simulink model "pmsm_foc_drive"  (R2021b)
settings: Solver=daessc  StartTime=0.0  StopTime=0.2  MaxStep=1e-3  RelTol=1e-3  AbsTol=1e-3  EnableMultiTasking=on
PreLoadFcn:
  | SystemParams;
StopFcn:
  | ee_addSimlogTimeStamp(bdroot)
undefined symbols (not defined in the file): ControllerParams, PmsmParams, SensorParams, TestScenarioParams
libraries: fl_lib x12, nesl_utility x8, ee_lib x2, spsFirstOrderFilterLib x1, simulink_extras x1
Description:
  | PMSM Drive Using Field-Oriented Control.
  | Copyright 2021 The MathWorks, Inc.
settings Model: Creator=agonzale  LastModifiedBy=agonzale
settings SolverCC: AutoScaleAbsTol=off  AlgebraicLoopSolver=TrustRegion
settings DataIOCC: LimitDataPoints=on  MaxDataPoints=10000
settings OptimizationCC: LifeSpan=inf
settings DebuggingCC: AllowSymbolicDim=off  SFUnexpectedBacktrackingDiag=warning  SFNoUnconditionalDefaultTransitionDiag=warning  SFExecutionAtInitializationDiag=none  SFMachineParentedDataDiag=warning  ArithmeticOperatorsInVariantConditions=warning
settings SFSimCC: SimUseLocalCustomCode=off  CustomCodeUndefinedFunction=UseInterfaceOnly
settings RTWCC: RTWUseLocalCustomCode=off
settings CodeAppCC: StateflowObjectComments=on
settings GRTTargetCC: TargetLangStandard=C89/C90 (ANSI)
settings ConfigComp: CovMetricSettings=dw  CovSaveCumulativeToWorkspaceVar=on  CovSaveSingleToWorkspaceVar=on  CovExternalEMLEnable=off  CovSFcnEnable=off
settings SimscapeCC: SimscapeLogType=all  SimscapeLogSimulationStatistics=on  SimscapeLogName=simlog_pmsm_foc_drive  SimscapeLogLimitData=off  SimscapeLogDataHistory=10000

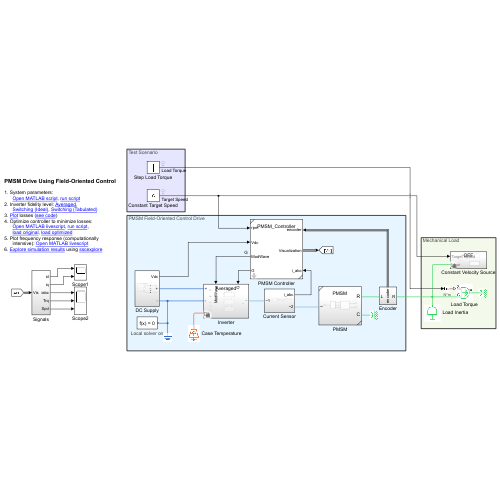
[thumbnail: Simulink's stored preview of the top-level diagram]
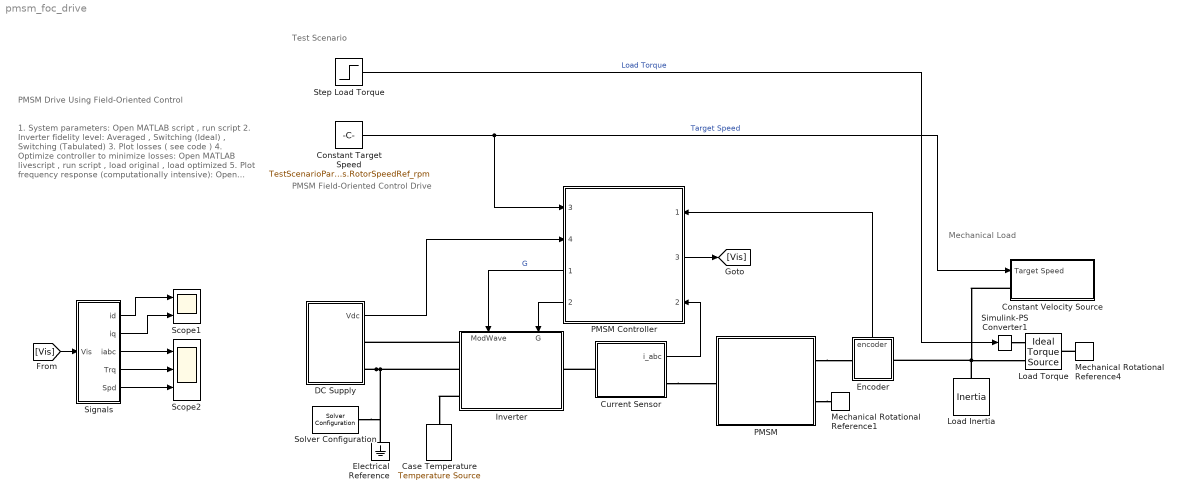
== system pmsm_foc_drive ==
  note: Mechanical Load
  note: PMSM Field-Oriented Control Drive
  note: Test Scenario
  note: 1. System parameters:
      | Open MATLAB script , run script
      | 2. Inverter fidelity level: Averaged ,
      | Switching (Ideal) , Switching (Tabulated)
      | 3. Plot losses ( see code )
      | 4. Optimize controller to minimize losses:
      | Open MATLAB livescript , run script ,
      | load original , load optimized
      | 5. Plot frequency response (computationally
      | intensive): Open MATLAB livescript
      | 6. Explore simulation results using sscexplore
  note: PMSM Drive Using Field-Oriented Control
  Case Temperature : fl_lib/Thermal/Thermal Sources/Temperature Source  temperature=InverterParams.TemperatureCase degC
  Constant Target Speed : Constant  Value=TestScenarioParams.RotorSpeedRef_rpm  SampleTime=ControllerParams.SampleTime
  Constant Velocity Source : Subsystem  Variant=on  VariantControlMode=label  LabelModeActiveChoice=OFF
  Current Sensor : Subsystem
  DC Supply : Subsystem
  Electrical Reference : fl_lib/Electrical/Electrical Elements/Electrical Reference
  Encoder : Subsystem
      settings: PortSchema="{\"entries\":[{\"content\":{\"sides\":[{\"content\":{\"connectorIds\":[\"LConn1\"]},\"type\":\"ConnectorPlacement.EquallySpacedRectSide\",\"uuid\":\"cfad22f7-4ca5-4e38-a161-f69c3faf7447\"},{\"content\":{\"connectorIds\":[\"RConn1\"],\"side\":\"RIGHT\"},\"type\":\"ConnectorPlacement.EquallySpacedRectSide\",\"uuid\":\"720e2ecf-f383-4111-97af-41d99d9b093d\"},{\"content\":{\"connectorIds\":[\"Out1\"],\"side\":\"TOP\"},\"type\":\"ConnectorPlacement.EquallySpacedRectSide\",\"uuid\":\"072894f0-fc0d-4f40-82e8-543eb6144e32\"}]},\"type\":\"ConnectorPlacement.EquallySpacedConnector\",\"uuid\":\"8d289e27-8023-447e-8610-dc73c3ce1339\"}],\"packageUris\":[\"http://schema.mathworks.com/mf0/Connector/R2020b\"],\"version\":\"1.0\"}"
  Inverter : Subsystem  Variant=on  VariantControlMode=label  VariantControl=Choice  LabelModeActiveChoice=Averaged
      settings: PortSchema="{\"entries\":[{\"content\":{\"sides\":[{\"content\":{\"connectorIds\":[\"LConn1\",\"LConn2\",\"LConn3\"]},\"type\":\"ConnectorPlacement.EquallySpacedRectSide\",\"uuid\":\"a5731130-aa3c-45df-b5d7-9e85c7611628\"},{\"content\":{\"connectorIds\":[\"RConn1\"],\"side\":\"RIGHT\"},\"type\":\"ConnectorPlacement.EquallySpacedRectSide\",\"uuid\":\"36730f5a-16d9-4cf3-b45d-c3a376589b1d\"},{\"content\":{\"connectorIds\":[\"In1\",\"In2\"],\"side\":\"TOP\"},\"type\":\"ConnectorPlacement.EquallySpacedRectSide\",\"uuid\":\"1e8f061d-b5bb-4e2a-be7e-dfb277e3f506\"}]},\"type\":\"ConnectorPlacement.EquallySpacedConnector\",\"uuid\":\"5a1efd64-0ec3-4b0f-b9d9-80575f7546cb\"}],\"packageUris\":[\"http://schema.mathworks.com/mf0/Connector/R2020b\"],\"version\":\"1.0\"}"
  Load Inertia : fl_lib/Mechanical/Rotational Elements/Inertia  inertia=MechLoadParams.Inertia kg*m^2  num_ports=foundation.enum.numPorts2.one  w_specify=on  w_priority=None  w=0 rpm  w_nominal_specify=off  w_nominal_unit=rad/s  w_nominal_value=1  t_specify=off  t_priority=None  t=0 N*m  t_nominal_specify=off  t_nominal_unit=N*m  t_nominal_value=1
  Load Torque : fl_lib/Mechanical/Mechanical Sources/Ideal Torque Source
  Mechanical Rotational Reference1 : fl_lib/Mechanical/Rotational Elements/Mechanical Rotational Reference
  Mechanical Rotational Reference4 : fl_lib/Mechanical/Rotational Elements/Mechanical Rotational Reference
  PMSM : Subsystem  ReferencedSubsystem=PMSM
  PMSM Controller : Subsystem  VariantControl=Averaged  ReferencedSubsystem=PMSM_Controller  ControllerParameters=ControllerParams
      settings: PortSchema="{\"entries\":[{\"content\":{\"sides\":[{\"content\":{\"connectorIds\":[\"In1\",\"Out3\",\"In2\"]},\"type\":\"ConnectorPlacement.EquallySpacedRectSide\",\"uuid\":\"4c32f1a4-bd89-4f05-8eaa-e2dd24abb257\"},{\"content\":{\"connectorIds\":[\"In3\",\"In4\",\"Out1\",\"Out2\"],\"side\":\"RIGHT\"},\"type\":\"ConnectorPlacement.EquallySpacedRectSide\",\"uuid\":\"3a536089-b16f-4be7-9641-6e190c11a3d2\"},{\"content\":{\"connectorIds\":[],\"side\":\"TOP\"},\"type\":\"ConnectorPlacement.EquallySpacedRectSide\",\"uuid\":\"a2701a3e-e366-4020-97eb-8b06a1d4835f\"}]},\"type\":\"ConnectorPlacement.EquallySpacedConnector\",\"uuid\":\"63f34eb4-489c-429c-82ff-74daaf150fe3\"}],\"packageUris\":[\"http://schema.mathworks.com/mf0/Connector/R2020b\"],\"version\":\"1.0\"}"
  Scope1 : Scope  NumInputPorts=2
  Scope2 : Scope  NumInputPorts=3
  "Signals " : Subsystem
  Simulink-PS Converter1 : nesl_utility/Simulink-PS Converter  PhysicalDomain=network_engine_domain  SubClassName=ps_input  LeftPortType=input  RightPortType=output  PseudoPeriodic=off  Frequencies=[]  NoiseDistribution=none  NoiseParameters=[]  Unit=N*m  AffineConversion=off  FilteringAndDerivatives=provide  SimscapeFilterOrder=1  InputFilterTimeConstant=0.001  UdotUserProvided=0
      settings: SourceProductBaseCode=PW,SS
  Solver Configuration : nesl_utility/Solver Configuration  Tag=ModelFeatures  PhysicalDomain=network_engine_domain  SubClassName=solver  LeftPortType=input  RightPortType=generic  Tones=[]  Harmonics=[]  SimulateNoise=off  Profile=off  UseLocalSampling=off  EnableSwitchedLinearOptims=on  FrequencyDomain=off  UseCCode=off  RelTol=0.001  AbsTol=1e-06  MinStep=1e-09  ToWorkspace=off  RevertToSquareIcSolve=off  NumHomotopyIterations=100  PhasorMode=off  PhasorModeNumHarmonics=1  DoDC=off  ResidualTolerance=1e-9  UseLocalSolver=on  LocalSolverChoice=NE_BACKWARD_EULER_ADVANCER  LocalSolverSampleTime=SolverParams.LocalSolverSampleTime  DoFixedCost=on  MaxNonlinIter=5  MaxModeIter=2  ComputeImpulses=off  ImpulseIterations=2  LinearAlgebra=auto  EquationFormulation=NE_TIME_EF  DelaysMemoryBudget=1024  AutomaticFiltering=on  FilteringTimeConstant=0.001  PartitionStorageMethod=AS_NEEDED  PartitionMemoryBudget=1024  PartitionMethod=FAST
      settings: AttributesFormatString=Local solver %<UseLocalSolver>  SourceProductBaseCode=PW,SS
  Step Load Torque : Step  Time=0.1  After=TestScenarioParams.StepTorqueAfter_Nm  SampleTime=0
  wires:
  Constant Target Speed/1 -> PMSM Controller/3, Constant Velocity Source/1(Target Speed)  "Target Speed"
  Step Load Torque/1 -> Simulink-PS Converter1/1  "Load Torque"
  [Vis] -> "Signals "/1(Vis)
  DC Supply/1(Vdc) -> PMSM Controller/4
  PMSM Controller/1 -> Inverter/1(ModWave)  "G"
  Encoder/1(encoder) -> PMSM Controller/1
  PMSM Controller/3 -> [Vis]
  Current Sensor/1(i_abc) -> PMSM Controller/2
  PMSM Controller/2 -> Inverter/2(G)
  "Signals "/1(id) -> Scope1/1
  "Signals "/2(iq) -> Scope1/2
  "Signals "/3(iabc) -> Scope2/1
  "Signals "/4(Trq) -> Scope2/2
  "Signals "/5(Spd) -> Scope2/3
  connections:
  Simulink-PS Converter1/RConn1 -- Load Torque/RConn1
  Mechanical Rotational Reference4/LConn1 -- Load Torque/LConn1
  DC Supply/RConn2 -- Inverter/LConn2 -- Electrical Reference/LConn1 -- Solver Configuration/RConn1
  Current Sensor/RConn1 -- PMSM/LConn1
  PMSM/RConn1 -- Encoder/LConn1
  Constant Velocity Source/LConn1 -- Load Torque/RConn2 -- Load Inertia/LConn1 -- Encoder/RConn1
  Inverter/LConn1 -- DC Supply/RConn1
  Current Sensor/LConn1 -- Inverter/RConn1
  Inverter/LConn3 -- Case Temperature/LConn1
  PMSM/RConn2 -- Mechanical Rotational Reference1/LConn1

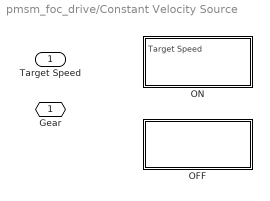
== system pmsm_foc_drive/Constant Velocity Source ==
  Target Speed : Inport
  OFF : Subsystem  VariantControl=OFF
  ON : Subsystem  VariantControl=ON
  Gear : PMIOPort  Side=Left

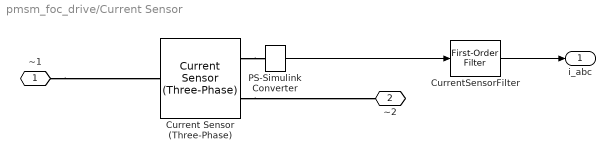
== system pmsm_foc_drive/Current Sensor ==
  Current Sensor (Three-Phase) : ee_lib/Sensors & Transducers/Current Sensor (Three-Phase)
  CurrentSensorFilter : spsFirstOrderFilterLib/First-Order Filter  FilterType=Lowpass  Tc=SensorParams.CurrentSensor.TimeConstant  Ts=0  Initialize=off  Vac_Init=[100, 0, 60]  Vdc_Init=0  PlotResponse=off  FreqRange="[0,  200,  1]"
  PS-Simulink Converter : nesl_utility/PS-Simulink Converter  PhysicalDomain=network_engine_domain  SubClassName=ps_output  LeftPortType=input  RightPortType=output  PseudoPeriodic=off  Frequencies=[]  Unit=A  AffineConversion=off
      settings: SourceProductBaseCode=PW,SS
  ~1 : PMIOPort  Side=Left
  ~2 : PMIOPort  Port=2  Side=Right
  i_abc : Outport
  wires:
  CurrentSensorFilter/1 -> i_abc/1
  PS-Simulink Converter/1 -> CurrentSensorFilter/1
  connections:
  ~1/RConn1 -- Current Sensor (Three-Phase)/LConn1
  Current Sensor (Three-Phase)/RConn1 -- PS-Simulink Converter/LConn1
  Current Sensor (Three-Phase)/RConn2 -- ~2/RConn1

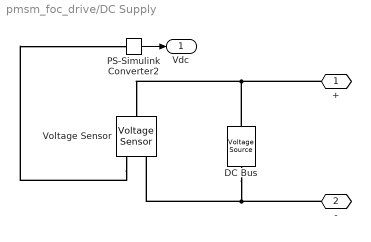
== system pmsm_foc_drive/DC Supply ==
  DC Bus : ee_lib/Sources/Voltage Source  dc_voltage=PowSupplyParams.DCVoltage_V V  ac_voltage=0 V  ac_shift=0 rad  ac_frequency=60 Hz  noise_mode=0  PSD=0 V^2/Hz  repeatability=1  auto_seed=4190380820  user_seed=0  sample_time=1e-3 s  i_specify=off  i_priority=None  i=0 A  i_nominal_specify=off  i_nominal_unit=A  i_nominal_value=1  v_specify=off  v_priority=None  v=0 V  v_nominal_specify=off  v_nominal_unit=V  v_nominal_value=1
  PS-Simulink Converter2 : nesl_utility/PS-Simulink Converter  PhysicalDomain=network_engine_domain  SubClassName=ps_output  LeftPortType=input  RightPortType=output  PseudoPeriodic=off  Frequencies=[]  Unit=V  AffineConversion=off
      settings: SourceProductBaseCode=PW,SS
  Voltage Sensor : fl_lib/Electrical/Electrical Sensors/Voltage Sensor
  + : PMIOPort  Side=Right
  - : PMIOPort  Port=2  Side=Right
  Vdc : Outport
  wires:
  PS-Simulink Converter2/1 -> Vdc/1
  connections:
  -/RConn1 -- DC Bus/RConn1 -- Voltage Sensor/RConn2
  Voltage Sensor/RConn1 -- PS-Simulink Converter2/LConn1
  +/RConn1 -- DC Bus/LConn1 -- Voltage Sensor/LConn1

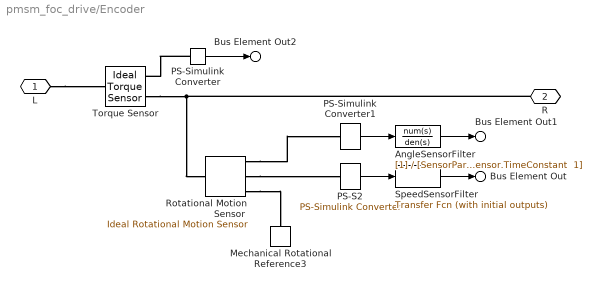
== system pmsm_foc_drive/Encoder ==
  AngleSensorFilter : TransferFcn  Denominator="[SensorParams.PositionSensor.TimeConstant  1]"
  Mechanical Rotational Reference3 : fl_lib/Mechanical/Rotational Elements/Mechanical Rotational Reference
  PS-S2 : nesl_utility/PS-Simulink Converter  PhysicalDomain=network_engine_domain  SubClassName=ps_output  LeftPortType=input  RightPortType=output  PseudoPeriodic=off  Frequencies=[]  Unit=rad/s  AffineConversion=off
      settings: SourceProductBaseCode=PW,SS
  PS-Simulink Converter : nesl_utility/PS-Simulink Converter  PhysicalDomain=network_engine_domain  SubClassName=ps_output  LeftPortType=input  RightPortType=output  PseudoPeriodic=off  Frequencies=[]  Unit=N*m  AffineConversion=off
      settings: SourceProductBaseCode=PW,SS
  PS-Simulink Converter1 : nesl_utility/PS-Simulink Converter  PhysicalDomain=network_engine_domain  SubClassName=ps_output  LeftPortType=input  RightPortType=output  PseudoPeriodic=off  Frequencies=[]  Unit=rad  AffineConversion=off
      settings: SourceProductBaseCode=PW,SS
  Rotational Motion Sensor : fl_lib/Mechanical/Mechanical Sensors/Ideal Rotational Motion Sensor  wrap_angle=simscape.enum.onoff.off  offset=0 rad
      settings: LogSimulationData=on
  SpeedSensorFilter : simulink_extras/Additional Linear/Transfer Fcn (with initial outputs)  N=[1]  D="[SensorParams.SpeedSensor.TimeConstant  1]"  Y0=PmsmParams.InitialRotorSpeed_rpm*2*pi/60  U0=0
  Torque Sensor : fl_lib/Mechanical/Mechanical Sensors/Ideal Torque Sensor
      settings: LogSimulationData=on
  L : PMIOPort  Side=Left
  R : PMIOPort  Port=2  Side=Right
  Bus Element Out : Outport  PortName=encoder  Element=w
      settings: AttributesFormatString=%<Unit>
  Bus Element Out1 : Outport  PortName=encoder  Element=a
      settings: AttributesFormatString=%<Unit>
  Bus Element Out2 : Outport  PortName=encoder  Element=trq
      settings: AttributesFormatString=%<Unit>
  wires:
  PS-S2/1 -> SpeedSensorFilter/1
  PS-Simulink Converter1/1 -> AngleSensorFilter/1
  AngleSensorFilter/1 -> Bus Element Out1/1
  SpeedSensorFilter/1 -> Bus Element Out/1
  PS-Simulink Converter/1 -> Bus Element Out2/1
  connections:
  Rotational Motion Sensor/RConn3 -- PS-Simulink Converter1/LConn1
  Rotational Motion Sensor/RConn2 -- PS-S2/LConn1
  R/RConn1 -- Torque Sensor/RConn1 -- Rotational Motion Sensor/LConn1
  L/RConn1 -- Torque Sensor/LConn1
  Rotational Motion Sensor/RConn1 -- Mechanical Rotational Reference3/LConn1
  PS-Simulink Converter/LConn1 -- Torque Sensor/RConn2

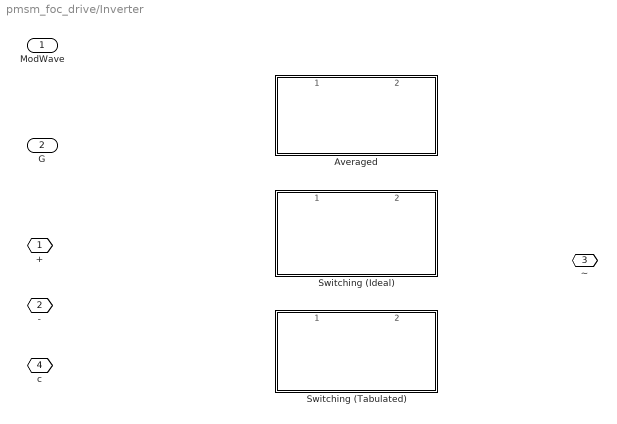
== system pmsm_foc_drive/Inverter ==
  ModWave : Inport
  G : Inport  Port=2
  Averaged : Subsystem  VariantControl=Averaged  ReferencedSubsystem=AveragedInverter
      settings: PortSchema="{\"entries\":[{\"content\":{\"sides\":[{\"content\":{\"connectorIds\":[\"LConn1\",\"LConn2\",\"LConn3\"]},\"type\":\"ConnectorPlacement.EquallySpacedRectSide\",\"uuid\":\"b77a7b87-9b1e-4a17-b6f6-338fca9d9cfe\"},{\"content\":{\"connectorIds\":[\"RConn1\"],\"side\":\"RIGHT\"},\"type\":\"ConnectorPlacement.EquallySpacedRectSide\",\"uuid\":\"84d00c63-1b9f-4e1b-a87e-6ae3bc20b0e8\"},{\"content\":{\"connectorIds\":[\"In1\",\"In2\"],\"side\":\"TOP\"},\"type\":\"ConnectorPlacement.EquallySpacedRectSide\",\"uuid\":\"34fb6523-0d29-4b30-bf80-8d7a8441c019\"}]},\"type\":\"ConnectorPlacement.EquallySpacedConnector\",\"uuid\":\"8748b1af-e44d-48ba-bbd0-c9117dbbd6f9\"}],\"packageUris\":[\"http://schema.mathworks.com/mf0/Connector/R2020b\"],\"version\":\"1.0\"}"
  Switching (Ideal) : Subsystem  VariantControl=Switching (Ideal)  ReferencedSubsystem=SwitchingInverterIdeal
      settings: PortSchema="{\"entries\":[{\"content\":{\"sides\":[{\"content\":{\"connectorIds\":[\"LConn1\",\"LConn2\",\"LConn3\"]},\"type\":\"ConnectorPlacement.EquallySpacedRectSide\",\"uuid\":\"b77a7b87-9b1e-4a17-b6f6-338fca9d9cfe\"},{\"content\":{\"connectorIds\":[\"RConn1\"],\"side\":\"RIGHT\"},\"type\":\"ConnectorPlacement.EquallySpacedRectSide\",\"uuid\":\"84d00c63-1b9f-4e1b-a87e-6ae3bc20b0e8\"},{\"content\":{\"connectorIds\":[\"In1\",\"In2\"],\"side\":\"TOP\"},\"type\":\"ConnectorPlacement.EquallySpacedRectSide\",\"uuid\":\"34fb6523-0d29-4b30-bf80-8d7a8441c019\"}]},\"type\":\"ConnectorPlacement.EquallySpacedConnector\",\"uuid\":\"8748b1af-e44d-48ba-bbd0-c9117dbbd6f9\"}],\"packageUris\":[\"http://schema.mathworks.com/mf0/Connector/R2020b\"],\"version\":\"1.0\"}"
  Switching (Tabulated) : Subsystem  VariantControl=Switching (Tabulated)  ReferencedSubsystem=SwitchingInverterTabulated
      settings: PortSchema="{\"entries\":[{\"content\":{\"sides\":[{\"content\":{\"connectorIds\":[\"LConn1\",\"LConn2\",\"LConn3\"]},\"type\":\"ConnectorPlacement.EquallySpacedRectSide\",\"uuid\":\"b77a7b87-9b1e-4a17-b6f6-338fca9d9cfe\"},{\"content\":{\"connectorIds\":[\"RConn1\"],\"side\":\"RIGHT\"},\"type\":\"ConnectorPlacement.EquallySpacedRectSide\",\"uuid\":\"84d00c63-1b9f-4e1b-a87e-6ae3bc20b0e8\"},{\"content\":{\"connectorIds\":[\"In1\",\"In2\"],\"side\":\"TOP\"},\"type\":\"ConnectorPlacement.EquallySpacedRectSide\",\"uuid\":\"34fb6523-0d29-4b30-bf80-8d7a8441c019\"}]},\"type\":\"ConnectorPlacement.EquallySpacedConnector\",\"uuid\":\"8748b1af-e44d-48ba-bbd0-c9117dbbd6f9\"}],\"packageUris\":[\"http://schema.mathworks.com/mf0/Connector/R2020b\"],\"version\":\"1.0\"}"
  + : PMIOPort  Tag=PMCPort  Side=Left
  - : PMIOPort  Tag=PMCPort  Port=2  Side=Left
  ~ : PMIOPort  Tag=PMCPort  Port=3  Side=Right
  c : PMIOPort  Tag=PMCPort  Port=4  Side=Left

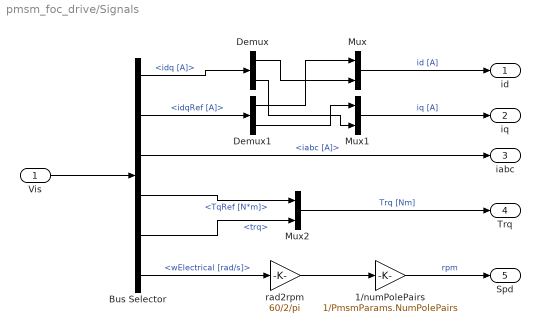
== system pmsm_foc_drive/Signals  ==
  Vis : Inport
  1/numPolePairs : Gain  Gain=1/PmsmParams.NumPolePairs
  Bus Selector : BusSelector  OutputSignals=Vis.idq [A],Vis.idqRef [A],Vis.iabc [A],Vis.TqRef [N*m],trq,Vis.wElectrical [rad/s]
  Demux : Demux  Outputs=2
  Demux1 : Demux  Outputs=2
  Mux : Mux  Inputs=2
  Mux1 : Mux  Inputs=2
  Mux2 : Mux  Inputs=2
  rad2rpm : Gain  Gain=60/2/pi
  id : Outport
  iq : Outport  Port=2
  iabc : Outport  Port=3  VectorParamsAs1DForOutWhenUnconnected=off
  Trq : Outport  Port=4  VectorParamsAs1DForOutWhenUnconnected=off
  Spd : Outport  Port=5  VectorParamsAs1DForOutWhenUnconnected=off
  wires:
  Vis/1 -> Bus Selector/1
  rad2rpm/1 -> 1/numPolePairs/1
  Bus Selector/1 -> Demux/1  "<idq [A]>"
  Bus Selector/2 -> Demux1/1  "<idqRef [A]>"
  1/numPolePairs/1 -> Spd/1  "rpm"
  Demux1/1 -> Mux/1
  Demux/1 -> Mux/2
  Demux1/2 -> Mux1/1
  Demux/2 -> Mux1/2
  Mux/1 -> id/1  "id [A]"
  Mux1/1 -> iq/1  "iq [A]"
  Bus Selector/3 -> iabc/1  "<iabc [A]>"
  Bus Selector/6 -> rad2rpm/1  "<wElectrical [rad/s]>"
  Bus Selector/4 -> Mux2/1  "<TqRef [N*m]>"
  Bus Selector/5 -> Mux2/2  "<trq>"
  Mux2/1 -> Trq/1  "Trq [Nm]"

== system pmsm_foc_drive/Constant Velocity Source/OFF ==

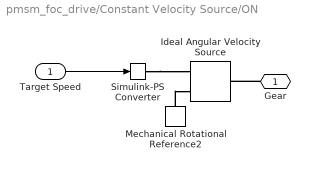
== system pmsm_foc_drive/Constant Velocity Source/ON ==
  Target Speed : Inport
  Ideal Angular Velocity Source : fl_lib/Mechanical/Mechanical Sources/Ideal Angular Velocity Source
  Mechanical Rotational Reference2 : fl_lib/Mechanical/Rotational Elements/Mechanical Rotational Reference
  Simulink-PS Converter : nesl_utility/Simulink-PS Converter  PhysicalDomain=network_engine_domain  SubClassName=ps_input  LeftPortType=input  RightPortType=output  PseudoPeriodic=off  Frequencies=[]  NoiseDistribution=none  NoiseParameters=[]  Unit=rpm  AffineConversion=off  FilteringAndDerivatives=provide  SimscapeFilterOrder=1  InputFilterTimeConstant=0.001  UdotUserProvided=0
      settings: SourceProductBaseCode=PW,SS
  Gear : PMIOPort  Side=Left
  wires:
  Target Speed/1 -> Simulink-PS Converter/1
  connections:
  Simulink-PS Converter/RConn1 -- Ideal Angular Velocity Source/RConn1
  Mechanical Rotational Reference2/LConn1 -- Ideal Angular Velocity Source/RConn2
  Gear/RConn1 -- Ideal Angular Velocity Source/LConn1
